simulink model "das2_inv"  (Simulink 6.4)
settings: Solver=ode4  StartTime=0.0  StopTime=0.25  MaxStep=0.001  RelTol=1e-3
undefined symbols (not defined in the file or in its folder): maxvel1, maxvel2, maxvel3, maxvel4, maxvel5, mu1, mu2, mu3, mu4, mu5
libraries: simulink x2
settings Model: Creator=chadwick  LastModifiedBy=Meg  ExtModeAutoUpdateStatusClock=off  BufferReuse=off  ProdHWDeviceType=32-bit xPC Target (Intel Pentium)
settings DataIOCC: MaxDataPoints=20000  SaveOutput=off  SignalLogging=off  SaveTime=off
settings OptimizationCC: BlockReduction=off  InlineParams=on  OptimizeBlockIOStorage=off  BufferReuse=off  ExpressionFolding=off  LocalBlockOutputs=off
settings HardwareCC: ProdIntDivRoundTo=Zero  ProdEndianess=LittleEndian  ProdHWDeviceType=32-bit xPC Target (Intel Pentium)
settings ModelReferenceCC: ModelReferenceNumInstancesAllowed=Single
settings RTWCC: SystemTargetFile=xpctarget.tlc  TemplateMakefile=xpc_default_tmf  Description=xPC Target  RetainRTWFile=on  ProcessScript=xpctarget_make_rtw_hook  CustomInclude=..\..\..\..\tools\sdbio\trunk\ ..\..\..\model\trunk\ ..\..\..\das1sim\trunk\  CustomSource=sdbio.c sdlib.c das1_d.c
settings xpcTargetCC: TargetFcnLib=ansi_tfl_tmw.mat  GenFloatMathFcnCalls=ANSI_C  IncludeERTFirstTime=on  RL32LogBufSizeModifier=1000

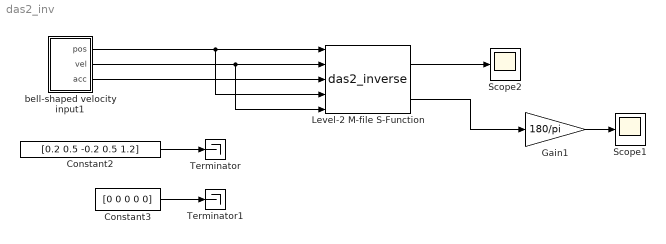
== system das2_inv ==
  Constant2 : Constant  Value=[0.2 0.5 -0.2 0.5 1.2]  OutDataType=sfix(16)  ConRadixGroup=Use specified scaling  OutScaling=2^0  SampleTime=0.002  FramePeriod=inf
  Constant3 : Constant  Value=[0 0 0 0 0]  OutDataType=sfix(16)  ConRadixGroup=Use specified scaling  OutScaling=2^0  SampleTime=0.002  FramePeriod=inf
  Gain1 : Gain  Gain=180/pi
  Level-2 M-file S-Function : M-S-Function  FunctionName=das2_inverse
  Scope1 : Scope
      settings: YMin=-40  YMax=80
  Scope2 : Scope
      settings: YMin=5.55112e-017  YMax=1  SaveName=act  DataFormat=Array
  Terminator : Terminator
  Terminator1 : Terminator
  bell-shaped velocity input1 : Subsystem
  wires:
  bell-shaped velocity input1/1(pos) -> Level-2 M-file S-Function/1, Level-2 M-file S-Function/4
  Gain1/1 -> Scope1/1
  Level-2 M-file S-Function/2 -> Gain1/1
  Level-2 M-file S-Function/1 -> Scope2/1
  bell-shaped velocity input1/2(vel) -> Level-2 M-file S-Function/2, Level-2 M-file S-Function/5
  bell-shaped velocity input1/3(acc) -> Level-2 M-file S-Function/3
  Constant2/1 -> Terminator/1
  Constant3/1 -> Terminator1/1

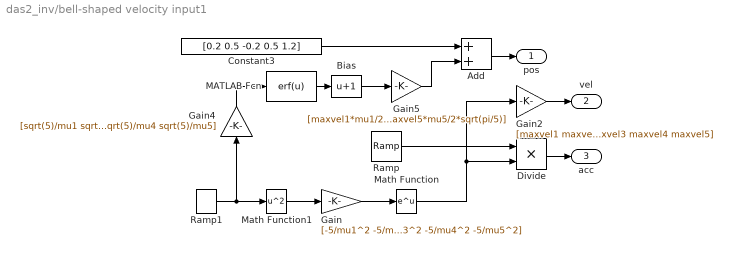
== system das2_inv/bell-shaped velocity input1 ==
  Add : Sum  OutScaling=2^-10
  Bias : Bias  Bias=1
  Constant3 : Constant  Value=[0.2 0.5 -0.2 0.5 1.2]  OutDataType=sfix(16)  ConRadixGroup=Use specified scaling  OutScaling=2^0  SampleTime=0.002  FramePeriod=inf
  Divide : Product  Inputs=**  OutScaling=2^-10
  Gain : Gain  Gain=[-5/mu1^2 -5/mu2^2 -5/mu3^2 -5/mu4^2 -5/mu5^2]
  Gain2 : Gain  Gain=[maxvel1 maxvel2 maxvel3 maxvel4 maxvel5]
  Gain4 : Gain  Orientation=up  Gain=[sqrt(5)/mu1 sqrt(5)/mu2 sqrt(5)/mu3 sqrt(5)/mu4 sqrt(5)/mu5]
  Gain5 : Gain  Gain=[maxvel1*mu1/2*sqrt(pi/5) maxvel2*mu2/2*sqrt(pi/5) maxvel3*mu3/2*sqrt(pi/5) maxvel4*mu4/2*sqrt(pi/5) maxvel5*mu5/2*sqrt(pi/5)]
  MATLAB Fcn : MATLABFcn  MATLABFcn=erf(u)
  Math Function : Math  SaturateOnIntegerOverflow=on
  Math Function1 : Math  Operator=square  SaturateOnIntegerOverflow=on
  Ramp : simulink/Sources/Ramp  SystemSampleTime=-1  slope=[-10*maxvel1/mu1^2 -10*maxvel2/mu2^2 -10*maxvel3/mu3^2 -10*maxvel4/mu4^2 -10*maxvel5/mu5^2]  start=0  X0=[10*maxvel1/mu1 10*maxvel2/mu2 10*maxvel3/mu3 10*maxvel4/mu4 10*maxvel5/mu5]
  Ramp1 : simulink/Sources/Ramp  SystemSampleTime=-1  slope=[1 1 1 1 1]  start=0  X0=[-mu1 -mu2 -mu3 -mu4 -mu5]
  pos : Outport
  vel : Outport  Port=2
  acc : Outport  Port=3
  wires:
  Ramp/1 -> Divide/1
  Math Function/1 -> Divide/2, Gain2/1
  Ramp1/1 -> Math Function1/1, Gain4/1
  Gain/1 -> Math Function/1
  Math Function1/1 -> Gain/1
  Gain4/1 -> MATLAB Fcn/1
  MATLAB Fcn/1 -> Bias/1
  Constant3/1 -> Add/1
  Bias/1 -> Gain5/1
  Gain5/1 -> Add/2
  Add/1 -> pos/1
  Gain2/1 -> vel/1
  Divide/1 -> acc/1
